simulink model "Exp2"  (R2025b)
settings: Solver=VariableStepAuto  StartTime=0.0  StopTime=10.0  RelTol=1e-3
libraries: commrandsrc3 x1, dspfdesign x1, dspsrcs4 x1
settings Model: Creator=pc  LastModifiedBy=pc

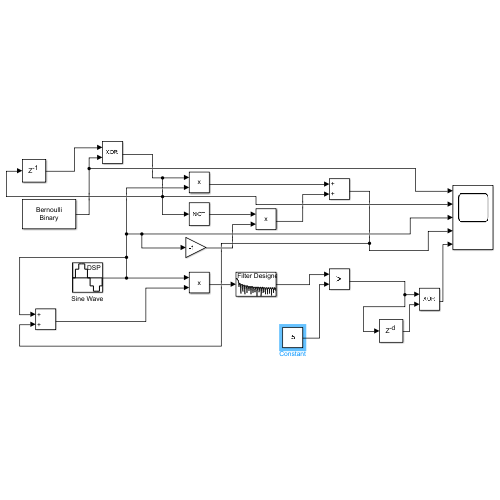
[thumbnail: Simulink's stored preview of the top-level diagram]
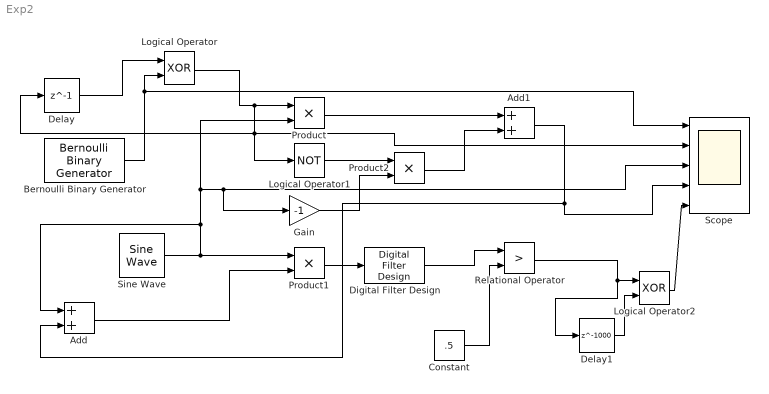
== system Exp2 ==
  Add : Sum
  Add1 : Sum
  Bernoulli Binary Generator : commrandsrc3/Bernoulli Binary Generator  ProbabilityOfZero=0.5  SeedSource=Auto  Seed=0  SampleTime=1  SamplesPerFrame=1  OutputDataType=double  SimulateUsing=Interpreted execution
  Constant : Constant  Value=.5
  Delay : Delay  DelayLength=1  InitialCondition=0
  Delay1 : Delay  DelayLength=1000  InitialCondition=0
  Digital Filter Design : dspfdesign/Digital Filter Design  mwdsp_browser_bugfix_var=off
  Gain : Gain  Gain=-1
  Logical Operator : Logic  Operator=XOR  AllPortsSameDT=off  OutDataTypeStr=boolean
  Logical Operator1 : Logic  Operator=NOT  AllPortsSameDT=off  OutDataTypeStr=boolean
  Logical Operator2 : Logic  Operator=XOR  AllPortsSameDT=off  OutDataTypeStr=boolean
  Product : Product
  Product1 : Product
  Product2 : Product
  Relational Operator : RelationalOperator  Operator=>  OutDataTypeStr=boolean  RndMeth=Simplest  InputSameDT=off
  Scope : Scope  NumInputPorts=5
      settings: ActiveDisplayYMinimum=-0.12499999999999997  ActiveDisplayYMaximum=1.125
  Sine Wave : dspsrcs4/Sine Wave  Amplitude=2  Frequency=5  Phase=0  SampleMode=Discrete  OutComplex=Real  CompMethod=Trigonometric fcn  TableSize=Speed  SampleTime=1/1000  SamplesPerFrame=1  ResetState=Restart at time zero  OutputFrames=off  dataType=double  wordLen=16  udDataType=sfix(16)  fracBitsMode=Best precision  numFracBits=15  OutDataTypeStr=double  LastOutDataTypeStr=double
  wires:
  Delay/1 -> Logical Operator/1
  Bernoulli Binary Generator/1 -> Scope/1, Logical Operator/2
  Logical Operator/1 -> Scope/2, Logical Operator1/1, Delay/1, Product/1
  Product/1 -> Add1/1
  Logical Operator1/1 -> Product2/1
  Gain/1 -> Product2/2
  Product2/1 -> Add1/2
  Add/1 -> Product1/2
  Product1/1 -> Digital Filter Design/1
  Digital Filter Design/1 -> Relational Operator/1
  Delay1/1 -> Logical Operator2/2
  Sine Wave/1 -> Add/1, Gain/1, Scope/3, Product/2, Product1/1
  Add1/1 -> Add/2, Scope/4
  Logical Operator2/1 -> Scope/5
  Constant/1 -> Relational Operator/2
  Relational Operator/1 -> Delay1/1, Logical Operator2/1
